simulink library "typhoonPatterns"  (R2017b)
settings: Solver=VariableStepAuto  StartTime=0.0  StopTime=10.0  RelTol=1e-3
undefined symbols (not defined in the file or in its folder): c_clamp, C_l, c_picoup_seq, crun_sp_ind, cst_sp_ind, f, f_picoup, f_sp_ind, fc, Jm, L, L1, L2, L_l, l_picoup_seq, La_DC, Ld, Lf_DC, Llr1_ind, Llr2_ind, Llr_ind, llrm_sp_ind, Lls_ind, llsa_sp_ind, llsm_sp_ind, Lm, Lq, n1, n2, nanm_sp_ind, pms, R, R1, R2, r_clamp, R_l, r_picoup_seq, Ra_DC, Rf_DC, Rm, Rr1_ind, Rr2_ind, Rr_ind, rrm_sp_ind, rrun_sp_ind, Rs, Rs_ind, rsa_sp_ind, rsm_sp_ind, rst_sp_ind
libraries: powerlib x282
(part 3 of 3)

== system typhoonPatterns/Symmetrical Boost ==
  gates : Inport
  Boost Converter : powerlib/Power Electronics/Boost Converter  ModelType=Switching devices  Ron=r_on  Rs=r_s  Cs=c_s  Vforward=[0, 0]  Ron_Diode=1e-3  Rs_Diode=1e6  Cs_Diode=inf  Vf_Diode=1e-3  Rs_CurrentSource=inf
      settings: SourceProductName=Simscape Power Systems  SourceProductBaseCode=PS
  Buck Converter : powerlib/Power Electronics/Buck Converter  ModelType=Switching devices  Ron=r_on  Rs=r_s  Cs=c_s  Vforward=[0, 0]  Ron_Diode=1e-3  Rs_Diode=1e6  Cs_Diode=inf  Vf_Diode=1e-3  Rs_CurrentSource=inf
      settings: SourceProductName=Simscape Power Systems  SourceProductBaseCode=PS
  Demux : Demux  Outputs=2
  inv1 : Logic  Commented=through  Operator=NOT  AllPortsSameDT=off  OutDataTypeStr=boolean
  inv2 : Logic  Commented=through  Operator=NOT  AllPortsSameDT=off  OutDataTypeStr=boolean
  In+ : PMIOPort  Port=1  Side=Left
  Out+ : PMIOPort  Port=2  Side=Right
  Out- : PMIOPort  Port=3  Side=Right
  In- : PMIOPort  Port=4  Side=Left
  wires:
  [S1] -> Boost Converter/1
  [S2] -> Buck Converter/1
  gates/1 -> Demux/1
  Demux/2 -> inv2/1
  Demux/1 -> inv1/1
  inv1/1 -> [S1]
  inv2/1 -> [S2]
  connections:
  In+/RConn1 -- Boost Converter/RConn1
  Buck Converter/RConn1 -- Boost Converter/RConn2
  Out+/RConn1 -- Boost Converter/LConn1
  Out-/RConn1 -- Buck Converter/RConn2
  In-/RConn1 -- Buck Converter/LConn1

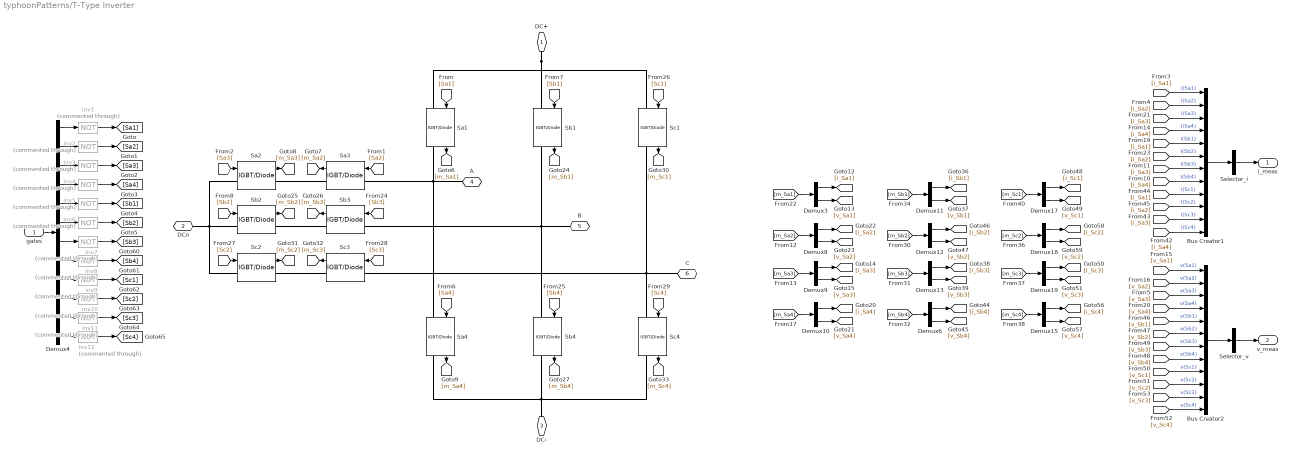
== system typhoonPatterns/T-Type Inverter ==
  gates : Inport
  Bus Creator1 : BusCreator  Inputs=12
  Bus Creator2 : BusCreator  Inputs=12
  Demux{3,6,8..13,15,17..19} (12 alike) : Demux  Outputs=2
  Demux4 : Demux  Outputs=12
  Sa{1..4} (4 alike) : powerlib/Power Electronics/IGBT//Diode  Ron=r_on  Rs=r_s  Cs=c_s  Measurements=on
  Sb{1..4} (4 alike) : powerlib/Power Electronics/IGBT//Diode  Ron=r_on  Rs=r_s  Cs=c_s  Measurements=on
  Sc{1..4} (4 alike) : powerlib/Power Electronics/IGBT//Diode  Ron=r_on  Rs=r_s  Cs=c_s  Measurements=on
  Selector_i : BusSelector  OutputSignals=i(Sa1)  OutputAsBus=on
  Selector_v : BusSelector  OutputSignals=v(Sa1)  OutputAsBus=on
  inv{1..12} (12 alike) : Logic  Commented=through  Operator=NOT  AllPortsSameDT=off  OutDataTypeStr=boolean
  DC+ : PMIOPort  Port=1  Side=Left
  DCn : PMIOPort  Port=2  Side=Left
  DC- : PMIOPort  Port=3  Side=Left
  A : PMIOPort  Port=4  Side=Right
  B : PMIOPort  Port=5  Side=Right
  C : PMIOPort  Port=6  Side=Right
  i_meas : Outport
  v_meas : Outport  Port=2
  wires:
  [v_Sc1] -> Bus Creator2/9  "v(Sc1)"
  [v_Sc2] -> Bus Creator2/10  "v(Sc2)"
  [v_Sc3] -> Bus Creator2/11  "v(Sc3)"
  [v_Sc4] -> Bus Creator2/12  "v(Sc4)"
  [v_Sb1] -> Bus Creator2/5  "v(Sb1)"
  [v_Sb2] -> Bus Creator2/6  "v(Sb2)"
  [v_Sb3] -> Bus Creator2/7  "v(Sb3)"
  [v_Sb4] -> Bus Creator2/8  "v(Sb4)"
  [i_Sa2] -> Bus Creator1/10  "i(Sc2)"
  [i_Sa3] -> Bus Creator1/11  "i(Sc3)"
  [i_Sa4] -> Bus Creator1/12  "i(Sc4)"
  [i_Sa1] -> Bus Creator1/9  "i(Sc1)"
  [i_Sa2] -> Bus Creator1/6  "i(Sb2)"
  [i_Sa3] -> Bus Creator1/7  "i(Sb3)"
  [i_Sa4] -> Bus Creator1/8  "i(Sb4)"
  [i_Sa1] -> Bus Creator1/5  "i(Sb1)"
  Demux17/1 -> [i_Sc1]
  Demux15/1 -> [i_Sc4]
  [m_Sc2] -> Demux18/1
  [m_Sc1] -> Demux17/1
  Demux19/1 -> [i_Sc3]
  Demux19/2 -> [v_Sc3]
  Demux17/2 -> [v_Sc1]
  Demux18/2 -> [v_Sc2]
  [m_Sc4] -> Demux15/1
  Demux15/2 -> [v_Sc4]
  Demux18/1 -> [i_Sc2]
  [m_Sc3] -> Demux19/1
  Demux11/1 -> [i_Sb1]
  Demux6/1 -> [i_Sb4]
  [m_Sb2] -> Demux12/1
  [m_Sb1] -> Demux11/1
  Demux13/1 -> [i_Sb3]
  Demux13/2 -> [v_Sb3]
  Demux11/2 -> [v_Sb1]
  Demux12/2 -> [v_Sb2]
  [m_Sb4] -> Demux6/1
  Demux6/2 -> [v_Sb4]
  Demux12/1 -> [i_Sb2]
  [m_Sb3] -> Demux13/1
  [Sc2] -> Sc2/1
  Sc1/1 -> [m_Sc1]
  Sc4/1 -> [m_Sc4]
  Sc2/1 -> [m_Sc2]
  [Sc1] -> Sc1/1
  Sc3/1 -> [m_Sc3]
  [Sc3] -> Sc3/1
  [Sc4] -> Sc4/1
  [Sb2] -> Sb2/1
  Sb1/1 -> [m_Sb1]
  Sb4/1 -> [m_Sb4]
  Sb2/1 -> [m_Sb2]
  [Sb1] -> Sb1/1
  Sb3/1 -> [m_Sb3]
  [Sb3] -> Sb3/1
  [Sb4] -> Sb4/1
  [Sa2] -> Sa3/1
  Sa1/1 -> [m_Sa1]
  Sa4/1 -> [m_Sa4]
  Sa3/1 -> [m_Sa2]
  [Sa1] -> Sa1/1
  Sa2/1 -> [m_Sa3]
  [Sa3] -> Sa2/1
  [Sa4] -> Sa4/1
  Selector_v/1 -> v_meas/1
  Demux3/1 -> [i_Sa1]
  [v_Sa4] -> Bus Creator2/4  "v(Sa4)"
  [v_Sa3] -> Bus Creator2/3  "v(Sa3)"
  [i_Sa4] -> Bus Creator1/4  "i(Sa4)"
  Demux3/2 -> [v_Sa1]
  Demux8/1 -> [i_Sa2]
  Bus Creator2/1 -> Selector_v/1
  [i_Sa1] -> Bus Creator1/1  "i(Sa1)"
  Demux9/2 -> [v_Sa3]
  Demux9/1 -> [i_Sa3]
  [v_Sa1] -> Bus Creator2/1  "v(Sa1)"
  Demux8/2 -> [v_Sa2]
  [i_Sa3] -> Bus Creator1/3  "i(Sa3)"
  Demux10/2 -> [v_Sa4]
  [m_Sa2] -> Demux8/1
  [m_Sa3] -> Demux9/1
  [m_Sa4] -> Demux10/1
  Demux10/1 -> [i_Sa4]
  Bus Creator1/1 -> Selector_i/1
  [v_Sa2] -> Bus Creator2/2  "v(Sa2)"
  Selector_i/1 -> i_meas/1
  [m_Sa1] -> Demux3/1
  [i_Sa2] -> Bus Creator1/2  "i(Sa2)"
  inv10/1 -> [Sc2]
  Demux4/11 -> inv11/1
  Demux4/12 -> inv12/1
  Demux4/7 -> inv7/1
  Demux4/8 -> inv8/1
  Demux4/9 -> inv9/1
  inv7/1 -> [Sb3]
  Demux4/10 -> inv10/1
  inv12/1 -> [Sc4]
  inv8/1 -> [Sb4]
  inv6/1 -> [Sb2]
  Demux4/6 -> inv6/1
  inv1/1 -> [Sa1]
  inv2/1 -> [Sa2]
  gates/1 -> Demux4/1
  Demux4/4 -> inv4/1
  Demux4/2 -> inv2/1
  Demux4/3 -> inv3/1
  Demux4/5 -> inv5/1
  inv4/1 -> [Sa4]
  Demux4/1 -> inv1/1
  inv9/1 -> [Sc1]
  inv5/1 -> [Sb1]
  inv11/1 -> [Sc3]
  inv3/1 -> [Sa3]
  connections:
  Sc4/RConn1 -- Sb4/RConn1 -- DC-/RConn1 -- Sa4/RConn1
  DC+/RConn1 -- Sc1/LConn1 -- Sb1/LConn1 -- Sa1/LConn1
  Sa2/RConn1 -- Sa3/RConn1
  Sb2/RConn1 -- Sb3/RConn1
  Sc2/RConn1 -- Sc3/RConn1
  Sa4/LConn1 -- A/RConn1 -- Sa3/LConn1 -- Sa1/RConn1
  Sb4/LConn1 -- Sb1/RConn1 -- B/RConn1 -- Sb3/LConn1
  Sc4/LConn1 -- Sc1/RConn1 -- C/RConn1 -- Sc3/LConn1
  Sa2/LConn1 -- DCn/RConn1 -- Sb2/LConn1 -- Sc2/LConn1

== system typhoonPatterns/TP 2W Transformer ==
  T1 : powerlib/Elements/Three-Phase Transformer (Two Windings)  Winding1Connection=Yg  Winding2Connection=Yg  CoreType=Three single-phase transformers  SetSaturation=off  Hysteresis=off  DataFile='hysteresis'  SetInitialFlux=off  Measurements=None  UNITS=SI  NominalPower=[1, 1]  Winding1=[1 1 1]  Winding2=[1 1 1]  Rm=1  Lm=1  L0=0.079577  Saturation=[0 0;0.0019596 0.15594;0.8165 0.19752]  InitialFluxes=[0.10396 -0.10396 0.090965]  MoreParameters=off  BreakLoop=off  DataType=on  TransfoNumber=1
      settings: AttributesFormatString=%<MaskType>
  prm_1 : PMIOPort  Port=1  Side=Left
  prm_2 : PMIOPort  Port=2  Side=Left
  prm_3 : PMIOPort  Port=3  Side=Left
  sec_1 : PMIOPort  Port=4  Side=Right
  sec_2 : PMIOPort  Port=5  Side=Right
  sec_3 : PMIOPort  Port=6  Side=Right
  connections:
  T1/LConn2 -- prm_2/RConn1
  T1/LConn1 -- prm_1/RConn1
  T1/LConn3 -- prm_3/RConn1
  sec_1/RConn1 -- T1/RConn1
  sec_2/RConn1 -- T1/RConn2
  sec_3/RConn1 -- T1/RConn3

== system typhoonPatterns/TP 3W Transformer ==
  T1 : powerlib/Elements/Three-Phase Transformer (Three Windings)  Winding1Connection=Y  Winding2Connection=Yg  Winding3Connection=Yg  CoreType=Three single-phase transformers  SetSaturation=off  Hysteresis=off  DataFile='hysteresis'  SetInitialFlux=off  Measurements=None  UNITS=SI  NominalPower=[1 , 1]  Winding1=[1 1 1]  Winding2=[1 1 1]  Winding3=[1 1 1]  Rm=1  Lm=1  L0=0.5  Saturation=[0 0;0.0019596 0.15594;0.8165 0.19752]  InitialFluxes=[0.10396 -0.10396 0.090965]  MoreParameters=off  BreakLoop=off  DataType=on  TransfoNumber=1
      settings: AttributesFormatString=%<MaskType>  SourceProductName=Simscape Power Systems  SourceProductBaseCode=PS
  prm_1 : PMIOPort  Port=1  Side=Left
  prm_2 : PMIOPort  Port=2  Side=Left
  prm_3 : PMIOPort  Port=3  Side=Left
  sec_1 : PMIOPort  Port=4  Side=Right
  sec_2 : PMIOPort  Port=5  Side=Right
  sec_3 : PMIOPort  Port=6  Side=Right
  sec_4 : PMIOPort  Port=7  Side=Right
  sec_5 : PMIOPort  Port=8  Side=Right
  sec_6 : PMIOPort  Port=9  Side=Right
  connections:
  T1/RConn3 -- sec_3/RConn1
  T1/RConn2 -- sec_2/RConn1
  T1/RConn1 -- sec_1/RConn1
  T1/LConn3 -- prm_3/RConn1
  T1/LConn1 -- prm_1/RConn1
  T1/LConn2 -- prm_2/RConn1
  T1/RConn6 -- sec_6/RConn1
  T1/RConn5 -- sec_5/RConn1
  T1/RConn4 -- sec_4/RConn1

== system typhoonPatterns/TP CC ==
  a_in : PMIOPort  Port=1  Side=Left
  b_in : PMIOPort  Port=2  Side=Left
  a_out : PMIOPort  Port=3  Side=Right
  b_out : PMIOPort  Port=4  Side=Right
  c_in : PMIOPort  Port=5  Side=Left
  c_out : PMIOPort  Port=6  Side=Right
  connections:
  a_in/RConn1 -- a_out/RConn1
  b_in/RConn1 -- b_out/RConn1
  c_in/RConn1 -- c_out/RConn1

== system typhoonPatterns/TPDT Contactor ==
  control : Inport
  Sa_1 : powerlib/Power Electronics/Ideal Switch  Ron=r_on  Lon=0  IC=s0  Rs=r_s  Cs=c_s  Measurements=on
  Sa_2 : powerlib/Power Electronics/Ideal Switch  Ron=r_on  Lon=0  IC=s0  Rs=r_s  Cs=c_s  Measurements=on
  Sb_1 : powerlib/Power Electronics/Ideal Switch  Ron=r_on  Lon=0  IC=s0  Rs=r_s  Cs=c_s  Measurements=on
  Sb_2 : powerlib/Power Electronics/Ideal Switch  Ron=r_on  Lon=0  IC=s0  Rs=r_s  Cs=c_s  Measurements=on
  Sc_1 : powerlib/Power Electronics/Ideal Switch  Ron=r_on  Lon=0  IC=s0  Rs=r_s  Cs=c_s  Measurements=on
  Sc_2 : powerlib/Power Electronics/Ideal Switch  Ron=r_on  Lon=0  IC=s0  Rs=r_s  Cs=c_s  Measurements=on
  inv1 : Logic  Commented=through  Operator=NOT  AllPortsSameDT=off  OutDataTypeStr=boolean
  inv2 : Logic  Operator=NOT  AllPortsSameDT=off  OutDataTypeStr=boolean
  A1 : PMIOPort  Port=1  Side=Left
  B1 : PMIOPort  Port=2  Side=Left
  C1 : PMIOPort  Port=3  Side=Right
  A2 : PMIOPort  Port=4  Side=Left
  B2 : PMIOPort  Port=5  Side=Left
  C2 : PMIOPort  Port=6  Side=Right
  A3 : PMIOPort  Port=7  Side=Left
  B3 : PMIOPort  Port=8  Side=Left
  C3 : PMIOPort  Port=9  Side=Right
  wires:
  [S_1] -> Sb_1/1
  [S_2] -> Sb_2/1
  inv1/1 -> inv2/1, [S_1]
  control/1 -> inv1/1
  inv2/1 -> [S_2]
  [S_1] -> Sa_1/1
  [S_2] -> Sa_2/1
  [S_2] -> Sc_2/1
  [S_1] -> Sc_1/1
  connections:
  B2/RConn1 -- Sb_2/LConn1
  A2/RConn1 -- Sb_1/LConn1
  Sb_1/RConn1 -- Sb_2/RConn1 -- C2/RConn1
  A1/RConn1 -- Sa_1/LConn1
  B1/RConn1 -- Sa_2/LConn1
  Sa_2/RConn1 -- C1/RConn1 -- Sa_1/RConn1
  C3/RConn1 -- Sc_1/RConn1 -- Sc_2/RConn1
  B3/RConn1 -- Sc_2/LConn1
  A3/RConn1 -- Sc_1/LConn1

== system typhoonPatterns/TPST Contactor ==
  control : Inport
  Sa : powerlib/Power Electronics/Ideal Switch  Ron=r_on  Lon=0  IC=s0  Rs=r_s  Cs=c_s  Measurements=on
  Sb : powerlib/Power Electronics/Ideal Switch  Ron=r_on  Lon=0  IC=s0  Rs=r_s  Cs=c_s  Measurements=on
  Sc : powerlib/Power Electronics/Ideal Switch  Ron=r_on  Lon=0  IC=s0  Rs=r_s  Cs=c_s  Measurements=on
  inv1 : Logic  Commented=through  Operator=NOT  AllPortsSameDT=off  OutDataTypeStr=boolean
  A1 : PMIOPort  Port=1  Side=Left
  B1 : PMIOPort  Port=2  Side=Right
  A2 : PMIOPort  Port=3  Side=Left
  B2 : PMIOPort  Port=4  Side=Right
  A3 : PMIOPort  Port=5  Side=Left
  B3 : PMIOPort  Port=6  Side=Right
  wires:
  inv1/1 -> [S]
  [S] -> Sb/1
  control/1 -> inv1/1
  [S] -> Sa/1
  [S] -> Sc/1
  connections:
  B2/RConn1 -- Sb/RConn1
  A1/RConn1 -- Sa/LConn1
  A2/RConn1 -- Sb/LConn1
  B1/RConn1 -- Sa/RConn1
  A3/RConn1 -- Sc/LConn1
  B3/RConn1 -- Sc/RConn1

== system typhoonPatterns/Thyristor Rectifier (1-Phase) ==
  gates : Inport
  Bus Creator : BusCreator  Inputs=4
  Bus Creator1 : BusCreator  Inputs=4
  Demux{1..3,5} (4 alike) : Demux  Outputs=2
  Demux4 : Demux
  Selector_i : BusSelector  OutputSignals=i(Sa_top)  OutputAsBus=on
  Selector_v : BusSelector  OutputSignals=v(Sa_top)  OutputAsBus=on
  inv{1..4} (4 alike) : Logic  Commented=through  Operator=NOT  AllPortsSameDT=off  OutDataTypeStr=boolean
  sa_bot : powerlib/Power Electronics/Thyristor  Ron=r_on  Lon=0  Vf=v_f  IC=0  Rs=r_s  Cs=c_s  Measurements=on
  sa_top : powerlib/Power Electronics/Thyristor  Ron=r_on  Lon=0  Vf=v_f  IC=0  Rs=r_s  Cs=c_s  Measurements=on
  sb_bot : powerlib/Power Electronics/Thyristor  Ron=r_on  Lon=0  Vf=v_f  IC=0  Rs=r_s  Cs=c_s  Measurements=on
  sb_top : powerlib/Power Electronics/Thyristor  Ron=r_on  Lon=0  Vf=v_f  IC=0  Rs=r_s  Cs=c_s  Measurements=on
  A : PMIOPort  Port=1  Side=Left
  B : PMIOPort  Port=2  Side=Left
  DC+ : PMIOPort  Port=3  Side=Right
  DC- : PMIOPort  Port=4  Side=Right
  i_meas : Outport
  v_meas : Outport  Port=2
  wires:
  inv4/1 -> [Sb_bot]
  sb_top/1 -> [m_Sb_top]
  [Sb_top] -> sb_top/1
  sa_bot/1 -> [m_Sa_bot]
  Demux4/4 -> inv4/1
  [Sa_top] -> sa_top/1
  Demux4/2 -> inv2/1
  inv2/1 -> [Sa_bot]
  [Sa_bot] -> sa_bot/1
  sb_bot/1 -> [m_Sb_bot]
  gates/1 -> Demux4/1
  inv3/1 -> [Sb_top]
  sa_top/1 -> [m_Sa_top]
  Demux4/3 -> inv3/1
  inv1/1 -> [Sa_top]
  [Sb_bot] -> sb_bot/1
  Demux4/1 -> inv1/1
  Demux2/2 -> [v_Sa_bot]
  Demux1/2 -> [v_Sa_top]
  [v_Sa_top] -> Bus Creator1/1  "v(Sa_top)"
  [i_Sb_top] -> Bus Creator/3  "i(Sb_top)"
  [i_Sb_bot] -> Bus Creator/4  "i(Sb_bot)"
  Demux5/2 -> [v_Sb_bot]
  Bus Creator1/1 -> Selector_v/1
  Demux3/2 -> [v_Sb_top]
  [v_Sb_bot] -> Bus Creator1/4  "v(Sb_bot)"
  Demux5/1 -> [i_Sb_bot]
  Selector_v/1 -> v_meas/1
  [v_Sb_top] -> Bus Creator1/3  "v(Sb_top)"
  [m_Sb_bot] -> Demux5/1
  [m_Sa_bot] -> Demux2/1
  Demux1/1 -> [i_Sa_top]
  [m_Sa_top] -> Demux1/1
  Bus Creator/1 -> Selector_i/1
  [m_Sb_top] -> Demux3/1
  Demux2/1 -> [i_Sa_bot]
  Selector_i/1 -> i_meas/1
  Demux3/1 -> [i_Sb_top]
  [v_Sa_bot] -> Bus Creator1/2  "v(Sa_bot)"
  [i_Sa_bot] -> Bus Creator/2  "i(Sa_bot)"
  [i_Sa_top] -> Bus Creator/1  "i(Sa_top)"
  connections:
  sa_top/RConn1 -- DC+/RConn1 -- sb_top/RConn1
  sa_bot/LConn1 -- DC-/RConn1 -- sb_bot/LConn1
  sa_bot/RConn1 -- sa_top/LConn1 -- A/RConn1
  sb_bot/RConn1 -- sb_top/LConn1 -- B/RConn1

== system typhoonPatterns/Thyristor Rectifier (3-Phase) ==
  gates : Inport
  Bus Creator1 : BusCreator  Inputs=6
  Bus Creator2 : BusCreator  Inputs=6
  Demux{1..3,8..10} (6 alike) : Demux  Outputs=2
  Demux4 : Demux  Outputs=6
  Selector_i : BusSelector  OutputSignals=i(Sa_top)  OutputAsBus=on
  Selector_v : BusSelector  OutputSignals=v(Sa_top)  OutputAsBus=on
  inv{1..6} (6 alike) : Logic  Commented=through  Operator=NOT  AllPortsSameDT=off  OutDataTypeStr=boolean
  sa_bot : powerlib/Power Electronics/Thyristor  Ron=r_on  Lon=0  Vf=v_f  IC=0  Rs=r_s  Cs=c_s  Measurements=on
  sa_top : powerlib/Power Electronics/Thyristor  Ron=r_on  Lon=0  Vf=v_f  IC=0  Rs=r_s  Cs=c_s  Measurements=on
  sb_bot : powerlib/Power Electronics/Thyristor  Ron=r_on  Lon=0  Vf=v_f  IC=0  Rs=r_s  Cs=c_s  Measurements=on
  sb_top : powerlib/Power Electronics/Thyristor  Ron=r_on  Lon=0  Vf=v_f  IC=0  Rs=r_s  Cs=c_s  Measurements=on
  sc_bot : powerlib/Power Electronics/Thyristor  Ron=r_on  Lon=0  Vf=v_f  IC=0  Rs=r_s  Cs=c_s  Measurements=on
  sc_top : powerlib/Power Electronics/Thyristor  Ron=r_on  Lon=0  Vf=v_f  IC=0  Rs=r_s  Cs=c_s  Measurements=on
  A : PMIOPort  Port=1  Side=Left
  B : PMIOPort  Port=2  Side=Left
  C : PMIOPort  Port=3  Side=Left
  DC+ : PMIOPort  Port=4  Side=Right
  DC- : PMIOPort  Port=5  Side=Right
  i_meas : Outport
  v_meas : Outport  Port=2
  wires:
  inv2/1 -> [Sa_bot]
  inv3/1 -> [Sb_top]
  Demux4/2 -> inv2/1
  inv1/1 -> [Sa_top]
  Demux4/1 -> inv1/1
  Demux4/3 -> inv3/1
  gates/1 -> Demux4/1
  Demux4/5 -> inv5/1
  inv6/1 -> [Sc_bot]
  Demux4/6 -> inv6/1
  inv4/1 -> [Sb_bot]
  inv5/1 -> [Sc_top]
  Demux4/4 -> inv4/1
  [Sa_top] -> sa_top/1
  [Sa_bot] -> sa_bot/1
  [Sb_top] -> sb_top/1
  [Sb_bot] -> sb_bot/1
  [Sc_top] -> sc_top/1
  [Sc_bot] -> sc_bot/1
  sa_top/1 -> [i_Sa_top]
  sa_bot/1 -> [i_Sa_bot]
  sb_top/1 -> [i_Sb_top]
  sb_bot/1 -> [i_Sb_bot]
  sc_top/1 -> [m_Sc_top]
  sc_bot/1 -> [i_Sc_bot]
  [i_Sa_bot] -> Bus Creator1/2  "i(Sa_bot)"
  Demux9/1 -> [i_Sb_top]
  Demux8/2 -> [v_Sa_bot]
  [m_Sa_top] -> Demux3/1
  Bus Creator1/1 -> Selector_i/1
  Demux9/2 -> [v_Sb_top]
  [m_Sc_bot] -> Demux1/1
  Bus Creator2/1 -> Selector_v/1
  Selector_v/1 -> v_meas/1
  [v_Sa_top] -> Bus Creator2/1  "v(Sa_top)"
  [i_Sb_bot] -> Bus Creator1/4  "i(Sb_bot)"
  [v_Sc_top] -> Bus Creator2/5  "v(Sc_top)"
  Demux2/2 -> [v_Sc_top]
  [i_Sb_top] -> Bus Creator1/3  "i(Sb_top)"
  [v_Sc_bot] -> Bus Creator2/6  "v(Sc_bot)"
  Demux10/2 -> [v_Sb_bot]
  Demux3/1 -> [i_Sa_top]
  [m_Sa_bot] -> Demux10/1
  Demux1/1 -> [i_Sc_bot]
  [i_Sc_top] -> Bus Creator1/5  "i(Sc_top)"
  [i_Sc_bot] -> Bus Creator1/6  "i(Sc_bot)"
  Demux3/2 -> [v_Sa_top]
  [m_Sc_top] -> Demux2/1
  [i_Sa_top] -> Bus Creator1/1  "i(Sa_top)"
  [m_Sb_top] -> Demux9/1
  Selector_i/1 -> i_meas/1
  [m_Sa_bot] -> Demux8/1
  [v_Sa_bot] -> Bus Creator2/2  "v(Sa_bot)"
  Demux1/2 -> [v_Sc_bot]
  Demux10/1 -> [i_Sb_bot]
  Demux2/1 -> [i_Sc_top]
  [v_Sb_top] -> Bus Creator2/3  "v(Sb_top)"
  [v_Sb_bot] -> Bus Creator2/4  "v(Sb_bot)"
  Demux8/1 -> [i_Sa_bot]
  connections:
  sa_bot/RConn1 -- sa_top/LConn1 -- A/RConn1
  sb_bot/RConn1 -- sb_top/LConn1 -- B/RConn1
  sc_bot/RConn1 -- sc_top/LConn1 -- C/RConn1
  sa_top/RConn1 -- DC+/RConn1 -- sc_top/RConn1 -- sb_top/RConn1
  sa_bot/LConn1 -- DC-/RConn1 -- sc_bot/LConn1 -- sb_bot/LConn1

== system typhoonPatterns/VSI (1-Phase) ==
  gates : Inport
  Bus Creator : BusCreator  Inputs=4
  Bus Creator1 : BusCreator  Inputs=4
  Demux{1..3,5} (4 alike) : Demux  Outputs=2
  Demux4 : Demux
  Selector_i : BusSelector  OutputSignals=i(Sa_top)  OutputAsBus=on
  Selector_v : BusSelector  OutputSignals=i(Sa_top)  OutputAsBus=on
  inv{1..4} (4 alike) : Logic  Commented=through  Operator=NOT  AllPortsSameDT=off  OutDataTypeStr=boolean
  sa_bot : powerlib/Power Electronics/IGBT//Diode  Ron=r_on  Rs=r_s  Cs=c_s  Measurements=on
  sa_top : powerlib/Power Electronics/IGBT//Diode  Ron=r_on  Rs=r_s  Cs=c_s  Measurements=on
  sb_bot : powerlib/Power Electronics/IGBT//Diode  Ron=r_on  Rs=r_s  Cs=c_s  Measurements=on
  sb_top : powerlib/Power Electronics/IGBT//Diode  Ron=r_on  Rs=r_s  Cs=c_s  Measurements=on
  A : PMIOPort  Port=1  Side=Right
  B : PMIOPort  Port=2  Side=Right
  DC+ : PMIOPort  Port=3  Side=Left
  DC- : PMIOPort  Port=4  Side=Left
  i_meas : Outport
  v_meas : Outport  Port=2
  wires:
  [i_Sa_top] -> Bus Creator/1  "i(Sa_top)"
  [i_Sa_bot] -> Bus Creator/2  "i(Sa_bot)"
  [v_Sa_bot] -> Bus Creator1/2  "v(Sa_bot)"
  Demux3/1 -> [i_Sb_top]
  Selector_i/1 -> i_meas/1
  Demux2/1 -> [i_Sa_bot]
  [m_Sb_top] -> Demux3/1
  Bus Creator/1 -> Selector_i/1
  [m_Sa_top] -> Demux1/1
  Demux1/1 -> [i_Sa_top]
  [m_Sa_bot] -> Demux2/1
  [m_Sb_bot] -> Demux5/1
  [v_Sb_top] -> Bus Creator1/3  "v(Sb_top)"
  Selector_v/1 -> v_meas/1
  Demux5/1 -> [i_Sb_bot]
  [v_Sb_bot] -> Bus Creator1/4  "v(Sb_bot)"
  Demux3/2 -> [v_Sb_top]
  Bus Creator1/1 -> Selector_v/1
  Demux5/2 -> [v_Sb_bot]
  [i_Sb_bot] -> Bus Creator/4  "i(Sb_bot)"
  [i_Sb_top] -> Bus Creator/3  "i(Sb_top)"
  [v_Sa_top] -> Bus Creator1/1  "v(Sa_top)"
  Demux1/2 -> [v_Sa_top]
  Demux2/2 -> [v_Sa_bot]
  Demux4/1 -> inv1/1
  inv1/1 -> [Sa_top]
  Demux4/3 -> inv3/1
  inv3/1 -> [Sb_top]
  gates/1 -> Demux4/1
  inv2/1 -> [Sa_bot]
  Demux4/2 -> inv2/1
  Demux4/4 -> inv4/1
  inv4/1 -> [Sb_bot]
  sa_top/1 -> [m_Sa_top]
  [Sa_top] -> sa_top/1
  sa_bot/1 -> [m_Sa_bot]
  [Sa_bot] -> sa_bot/1
  sb_bot/1 -> [m_Sb_bot]
  [Sb_bot] -> sb_bot/1
  sb_top/1 -> [m_Sb_top]
  [Sb_top] -> sb_top/1
  connections:
  DC-/RConn1 -- sb_bot/RConn1 -- sa_bot/RConn1
  sa_top/RConn1 -- A/RConn1 -- sa_bot/LConn1
  sb_top/RConn1 -- B/RConn1 -- sb_bot/LConn1
  DC+/RConn1 -- sb_top/LConn1 -- sa_top/LConn1

== system typhoonPatterns/VSI (3-Phase) ==
  gates : Inport
  Bus Creator1 : BusCreator  Inputs=6
  Bus Creator2 : BusCreator  Inputs=6
  Demux{1..3,8..10} (6 alike) : Demux  Outputs=2
  Demux4 : Demux  Outputs=6
  Selector_i : BusSelector  OutputSignals=i(Sa_top)  OutputAsBus=on
  Selector_v : BusSelector  OutputSignals=v(Sa_top)  OutputAsBus=on
  inv{1..6} (6 alike) : Logic  Commented=through  Operator=NOT  AllPortsSameDT=off  OutDataTypeStr=boolean
  sa_bot : powerlib/Power Electronics/IGBT//Diode  Ron=r_on  Rs=r_s  Cs=c_s  Measurements=on
  sa_top : powerlib/Power Electronics/IGBT//Diode  Ron=r_on  Rs=r_s  Cs=c_s  Measurements=on
  sb_bot : powerlib/Power Electronics/IGBT//Diode  Ron=r_on  Rs=r_s  Cs=c_s  Measurements=on
  sb_top : powerlib/Power Electronics/IGBT//Diode  Ron=r_on  Rs=r_s  Cs=c_s  Measurements=on
  sc_bot : powerlib/Power Electronics/IGBT//Diode  Ron=r_on  Rs=r_s  Cs=c_s  Measurements=on
  sc_top : powerlib/Power Electronics/IGBT//Diode  Ron=r_on  Rs=r_s  Cs=c_s  Measurements=on
  A : PMIOPort  Port=1  Side=Right
  B : PMIOPort  Port=2  Side=Right
  DC+ : PMIOPort  Port=3  Side=Left
  DC- : PMIOPort  Port=4  Side=Left
  C : PMIOPort  Port=5  Side=Right
  i_meas : Outport
  v_meas : Outport  Port=2
  wires:
  inv2/1 -> [Sa_bot]
  inv3/1 -> [Sb_top]
  Demux4/2 -> inv2/1
  inv1/1 -> [Sa_top]
  Demux4/1 -> inv1/1
  Demux4/3 -> inv3/1
  gates/1 -> Demux4/1
  Demux4/5 -> inv5/1
  inv6/1 -> [Sc_bot]
  Demux4/6 -> inv6/1
  inv4/1 -> [Sb_bot]
  inv5/1 -> [Sc_top]
  Demux4/4 -> inv4/1
  sa_top/1 -> [m_Sa_top]
  sb_bot/1 -> [m_Sb_bot]
  [Sb_top] -> sb_top/1
  sa_bot/1 -> [m_Sa_bot]
  sb_top/1 -> [m_Sb_top]
  [Sb_bot] -> sb_bot/1
  [Sa_top] -> sa_top/1
  [Sa_bot] -> sa_bot/1
  sc_top/1 -> [m_Sc_top]
  sc_bot/1 -> [m_Sc_bot]
  [Sc_top] -> sc_top/1
  [Sc_bot] -> sc_bot/1
  [i_Sa_bot] -> Bus Creator1/2  "i(Sa_bot)"
  Demux9/1 -> [i_Sb_top]
  Demux8/2 -> [v_Sa_bot]
  [m_Sa_top] -> Demux3/1
  Bus Creator1/1 -> Selector_i/1
  Demux9/2 -> [v_Sb_top]
  [m_Sc_bot] -> Demux1/1
  Bus Creator2/1 -> Selector_v/1
  Selector_v/1 -> v_meas/1
  [v_Sa_top] -> Bus Creator2/1  "v(Sa_top)"
  [i_Sb_bot] -> Bus Creator1/4  "i(Sb_bot)"
  [v_Sc_top] -> Bus Creator2/5  "v(Sc_top)"
  Demux2/2 -> [v_Sc_top]
  [i_Sb_top] -> Bus Creator1/3  "i(Sb_top)"
  [v_Sc_bot] -> Bus Creator2/6  "v(Sc_bot)"
  Demux10/2 -> [v_Sb_bot]
  Demux3/1 -> [i_Sa_top]
  [m_Sb_bot] -> Demux10/1
  Demux1/1 -> [i_Sc_bot]
  [i_Sc_top] -> Bus Creator1/5  "i(Sc_top)"
  [i_Sc_bot] -> Bus Creator1/6  "i(Sc_bot)"
  Demux3/2 -> [v_Sa_top]
  [m_Sc_top] -> Demux2/1
  [i_Sa_top] -> Bus Creator1/1  "i(Sa_top)"
  [m_Sb_top] -> Demux9/1
  Selector_i/1 -> i_meas/1
  [m_Sa_bot] -> Demux8/1
  [v_Sa_bot] -> Bus Creator2/2  "v(Sa_bot)"
  Demux1/2 -> [v_Sc_bot]
  Demux10/1 -> [i_Sb_bot]
  Demux2/1 -> [i_Sc_top]
  [v_Sb_top] -> Bus Creator2/3  "v(Sb_top)"
  [v_Sb_bot] -> Bus Creator2/4  "v(Sb_bot)"
  Demux8/1 -> [i_Sa_bot]
  connections:
  sa_bot/RConn1 -- sc_bot/RConn1 -- sb_bot/RConn1 -- DC-/RConn1
  sa_bot/LConn1 -- A/RConn1 -- sa_top/RConn1
  sb_bot/LConn1 -- B/RConn1 -- sb_top/RConn1
  sa_top/LConn1 -- sc_top/LConn1 -- sb_top/LConn1 -- DC+/RConn1
  sc_bot/LConn1 -- C/RConn1 -- sc_top/RConn1

== system typhoonPatterns/Vienna Rectifier ==
  gates : Inport
  Bus Creator1 : BusCreator  Inputs=3
  Bus Creator2 : BusCreator  Inputs=3
  D{1..6} (6 alike) : powerlib/Power Electronics/Diode  Ron=r_on  Lon=0  Vf=v_f  IC=0  UseSnubber=0  Rs=r_s  Cs=c_s  Measurements=off
  Demux : Demux  Outputs=3
  Demux6 : Demux  Outputs=2
  Demux8 : Demux  Outputs=2
  Demux9 : Demux  Outputs=2
  Diode Bridge : powerlib/Power Electronics/Universal Bridge  Arms=2  SnubberResistance=r_s  SnubberCapacitance=c_s  Device=Diodes  Ron=r_on  Lon=0  ForwardVoltages="[  0  0  ]"  ForwardVoltage=v_f  GTOparameters=[ 10e-6 , 20e-6 ]  IGBTparameters=[ 1e-6 , 2e-6 ]  Measurements=None  Measurements_2=None  converterType=Rectifier
  Diode Bridge1 : powerlib/Power Electronics/Universal Bridge  Arms=2  SnubberResistance=r_s  SnubberCapacitance=c_s  Device=Diodes  Ron=r_on  Lon=0  ForwardVoltages="[  0  0  ]"  ForwardVoltage=v_f  GTOparameters=[ 10e-6 , 20e-6 ]  IGBTparameters=[ 1e-6 , 2e-6 ]  Measurements=None  Measurements_2=None  converterType=Rectifier
  Diode Bridge2 : powerlib/Power Electronics/Universal Bridge  Arms=2  SnubberResistance=r_s  SnubberCapacitance=c_s  Device=Diodes  Ron=r_on  Lon=0  ForwardVoltages="[  0  0  ]"  ForwardVoltage=v_f  GTOparameters=[ 10e-6 , 20e-6 ]  IGBTparameters=[ 1e-6 , 2e-6 ]  Measurements=None  Measurements_2=None  converterType=Rectifier
  S_a : powerlib/Power Electronics/IGBT  Ron=r_on  Lon=0  Vf=v_f  Tf=1e-6  Tt=2e-6  IC=0  Rs=r_s  Cs=c_s  Measurements=on
  S_b : powerlib/Power Electronics/IGBT  Ron=r_on  Lon=0  Vf=v_f  Tf=1e-6  Tt=2e-6  IC=0  Rs=r_s  Cs=c_s  Measurements=on
  S_c : powerlib/Power Electronics/IGBT  Ron=r_on  Lon=0  Vf=v_f  Tf=1e-6  Tt=2e-6  IC=0  Rs=r_s  Cs=c_s  Measurements=on
  Selector_i : BusSelector  OutputSignals=i(Sa)  OutputAsBus=on
  Selector_v : BusSelector  OutputSignals=v(Sa)  OutputAsBus=on
  inv1 : Logic  Commented=through  Operator=NOT  AllPortsSameDT=off  OutDataTypeStr=boolean
  inv2 : Logic  Commented=through  Operator=NOT  AllPortsSameDT=off  OutDataTypeStr=boolean
  inv3 : Logic  Commented=through  Operator=NOT  AllPortsSameDT=off  OutDataTypeStr=boolean
  A : PMIOPort  Port=1  Side=Left
  B : PMIOPort  Port=2  Side=Left
  C : PMIOPort  Port=3  Side=Left
  DC+ : PMIOPort  Port=4  Side=Right
  DCn : PMIOPort  Port=5  Side=Right
  DC- : PMIOPort  Port=6  Side=Right
  i_meas : Outport
  v_meas : Outport  Port=2
  wires:
  gates/1 -> Demux/1
  Demux/1 -> inv1/1
  Demux/2 -> inv2/1
  Demux/3 -> inv3/1
  [Sa] -> S_a/1
  [Sb] -> S_b/1
  [Sc] -> S_c/1
  inv1/1 -> [Sa]
  inv2/1 -> [Sb]
  inv3/1 -> [Sc]
  S_a/1 -> [m_Sa]
  S_b/1 -> [m_Sb]
  S_c/1 -> [m_Sc]
  [m_Sa] -> Demux6/1
  Demux9/1 -> [i_Sc]
  [i_Sa] -> Bus Creator1/1  "i(Sa)"
  Bus Creator1/1 -> Selector_i/1
  [v_Sb] -> Bus Creator2/2  "v(Sb)"
  Selector_i/1 -> i_meas/1
  Selector_v/1 -> v_meas/1
  Demux8/2 -> [v_Sb]
  Demux6/2 -> [v_Sa]
  [i_Sc] -> Bus Creator1/3  "i(Sc)"
  Demux8/1 -> [i_Sb]
  [v_Sc] -> Bus Creator2/3  "v(Sc)"
  Bus Creator2/1 -> Selector_v/1
  [i_Sb] -> Bus Creator1/2  "i(Sb)"
  Demux6/1 -> [i_Sa]
  [m_Sc] -> Demux9/1
  [v_Sa] -> Bus Creator2/1  "v(Sa)"
  Demux9/2 -> [v_Sc]
  [m_Sb] -> Demux8/1
  connections:
  D1/LConn1 -- S_a/LConn1 -- Diode Bridge/RConn1
  D2/RConn1 -- Diode Bridge/RConn2 -- S_a/RConn1
  Diode Bridge1/RConn2 -- S_b/RConn1 -- D4/RConn1
  Diode Bridge1/RConn1 -- S_b/LConn1 -- D3/LConn1
  Diode Bridge2/RConn2 -- S_c/RConn1 -- D6/RConn1
  Diode Bridge2/RConn1 -- S_c/LConn1 -- D5/LConn1
  Diode Bridge2/LConn1 -- C/RConn1
  Diode Bridge/LConn1 -- A/RConn1
  Diode Bridge1/LConn1 -- B/RConn1
  Diode Bridge/LConn2 -- DCn/RConn1 -- Diode Bridge2/LConn2 -- Diode Bridge1/LConn2
  D1/RConn1 -- DC+/RConn1 -- D5/RConn1 -- D3/RConn1
  D4/LConn1 -- D6/LConn1 -- DC-/RConn1 -- D2/LConn1
